simulink model "purePursuitUSCity"  (R2022b)
settings: Solver=VariableStepAuto  StartTime=0.0  StopTime=Ts  RelTol=1e-3
PreLoadFcn:
  | setUpPurePursuitUSCity
model workspace (MAT data in the model file):
  firstWarning = 0
  originalScenarioChecksum = 'F73A6DA3C723D3CA73A6F931B7A52A9C'
values from neighbouring files (symbols this model uses):
  diffcurve = []    [setUpPurePursuitUSCity.m]
  L = data.ActorSpecifications.Length    [setUpPurePursuitUSCity.m]
  ld = 5    [setUpPurePursuitUSCity.m]
  psi_o = refPose(1,3)    [setUpPurePursuitUSCity.m]
  s = size(xRef)    [setUpPurePursuitUSCity.m]
  X_o = refPose(1,1)    [setUpPurePursuitUSCity.m]
  xRef = refPose(:,1)    [setUpPurePursuitUSCity.m]
  Y_o = -refPose(1,2)    [setUpPurePursuitUSCity.m]
  yRef = -refPose(:,2)    [setUpPurePursuitUSCity.m]
undefined symbols (not defined in the file or in its folder): data, deg, rad
libraries: autolibutils x4, autolibshared x3, vehdynlibviscommon x1, aerolibconvert2 x1, simulink_extras x1, drivingscenarioandsensors x1, robotalgslib x1, simulink x1, sim3dlib x1, vdynlib x1
(part 1 of 3)
settings Model: PacingRate=0.700000  Creator=valakshe  LastModifiedBy=burak
settings SolverCC: AlgebraicLoopSolver=TrustRegion
settings DebuggingCC: UnconnectedInputMsg=warning  UnconnectedOutputMsg=warning  UnconnectedLineMsg=warning  SFMachineParentedDataDiag=warning
settings ModelReferenceCC: EnableRefExpFcnMdlSchedulingChecks=on
settings RTWCC: DLArmComputeVersion=19.05

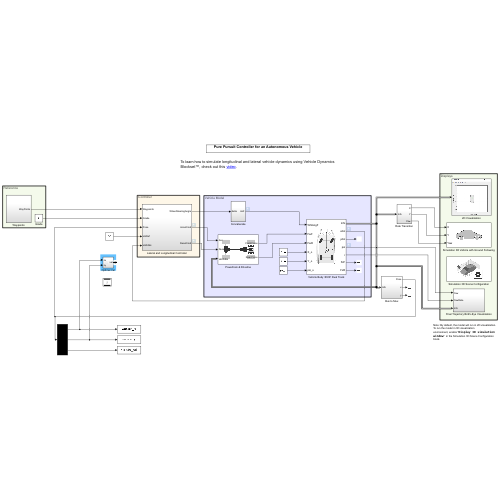
[thumbnail: Simulink's stored preview of the top-level diagram]
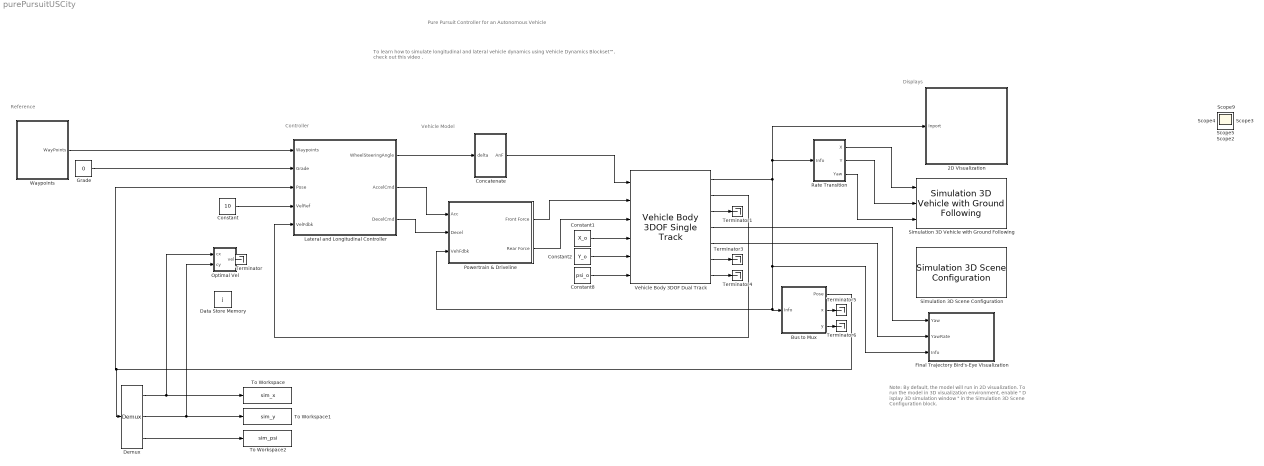
== system purePursuitUSCity ==
  note: Note: By default, the model will run in 2D visualization. To run the model in 3D visualization
      | environment, enable " D isplay 3D simulation window " in the Simulation 3D Scene Configuration block.
  note: To learn how to simulate longitudinal and lateral vehicle dynamics using Vehicle Dynamics
      | Blockset™, check out this video .
  note: Pure Pursuit Controller for an Autonomous Vehicle
  note: Reference
  note: Controller
  note: Vehicle Model
  note: Displays
  2D Visualization : Subsystem
      mask Display: image("visualization.JPG");
  Bus to Mux : Subsystem
  Concatenate : Subsystem
  Constant : Constant  Value=10
  Constant1 : Constant  Value=X_o
  Constant2 : Constant  Value=Y_o
  Constant8 : Constant  Value=psi_o
  Data Store Memory : DataStoreMemory  DataStoreName=j  WriteAfterWriteMsg=warning  InitialValue=j  ShowAdditionalParam=off
  Demux : Demux  Outputs=3
  Final Trajectory Bird's-Eye Visualization : Subsystem
  Grade : Constant  Value=0
  Lateral and Longitudinal Controller : Subsystem
  Optimal Vel : Subsystem
  Powertrain & Driveline : Subsystem
      mask Display: image('vdbslibpt.png');
  Rate Transition : Subsystem
  Simulation 3D Scene Configuration : sim3dlib/Simulation 3D Scene Configuration  Priority=1  ProjectFormat=Default Scenes  SceneDesc=Curved road  ProjectName=C:\Program Files\MATLAB\R2022b\toolbox\shared\sim3d_projects\automotive_project\UE4\WindowsNoEditor\VehicleSimulation.exe  ScenePath=8mile  UEProjPath=C:\Local\AutoVrtlEnv\AutoVrtlEnv.uproject  EnableOpenDRIVE=off  vehTagList={'Scene Origin';'SimulinkVehicle1'}  vehTag=SimulinkVehicle1  OpVisEn=off  Ts=.05  EnableWindow=on  EnableRemoteAccess=off  EnableWeather=off  SunAltitude=40.0  SunAzimuth=90  clouds=10  wind=1  fog=0  rain=0  EnableGeospatial=off  OriginHeight=200  OriginLatitude=40.744652  OriginLongitude=-73.988864  MapStyle=Aerial  AdditionalAssetIDs=[]  UseAdvancedSunSky=off  SolarTime=11  TimeZone=-5  Day=21  Month=9  Year=2022  UseDaylightSavingTime=on  DSTStartDay=10  DSTStartMonth=3  DSTEndDay=3  DSTEndMonth=11  DSTSwitchHour=2  sensorTag=MainCamera1  sensorId=1  sensorName=MainCamera1  mountLoc=Origin  offsetFlag=off  tmountOffset=[0, 0, 0]  rmountOffset=[0, 0, 0]  HorizontalResolution=1280  VerticalResolution=720  HorizontalFOV=60  mountPoint=[0 0 0]  mountOrientation=[0 0 0]  aMode=2  ID=1  GeoTrigger=Inactive
  Simulation 3D Vehicle with Ground Following : vdynlib/Vehicle Scenarios/Sim3D/Sim3D Vehicle/Components/Simulation 3D Vehicle with Ground Following  Priority=-1  PassVehMesh=Muscle car  MeshPath=/MathWorksSimulation/Vehicles/Muscle/Meshes/SK_MuscleCar.SK_MuscleCar  TrackWidth=1.9  WheelBase=3  WheelRadius=0.35  VehColor=Yellow  InitialPos=[0,0,0]  InitialRot=[0, 0, 0]  ActorName=SimulinkVehicle1  VehLightsControl=off  HeadlightColor=[ 1, 1, 1 ]  HighBeamIntensity=100000  LowBeamIntensity=60000  HighBeamConeAngle=1.22  LowBeamConeAngle=1.22  LeftHeadlightOrientation=[ 0, 0 ]  RightHeadlightOrientation=[ 0, 0 ]  BrakelightIntensity=200  ReverselightIntensity=500  SignallightIntensity=500  SignallightPeriod=1  SignalPulseWidth=50  SampleTime=-1  ActorType=SimulinkVehicle  ID=1  aMode=2  ActorTag=SimulinkVehicle1  CoordinateScheme=SAE
  Terminator{,1,3..6} (6 alike) : Terminator
  To Workspace : ToWorkspace  VariableName=sim_x  SaveFormat=Timeseries  SampleTime=-1
  To Workspace1 : ToWorkspace  VariableName=sim_y  SaveFormat=Timeseries  SampleTime=-1
  To Workspace2 : ToWorkspace  VariableName=sim_psi  SaveFormat=Timeseries  SampleTime=-1
  Vehicle Body 3DOF Dual Track : autolibshared/Vehicle Body 3DOF Single Track  trackMode=Dual  inputMode=External longitudinal forces  frontSteerMode=on  rearSteerMode=off  windMode=off  muMode=off  extFMode=off  extMMode=off  htchFMode=off  htchMMode=off  extXo=on  extpsio=on  extxdoto=off  extro=off  extYo=on  extTamb=off  extydoto=off  aMode=2  NF=2  NR=2  m=2000  a=1.4  b=1.6  h=0.35  dh=1  hh=0.2  X_o=0  xdot_o=0  CalphaMode=off  sigmaMode=on  d=0  hl=0  w=[1.4,1.4]  Cy_f=12e3  Cy_r=11e3  sigma_f=.1  sigma_r=.1  alpha_f_brk=[-.1 .1]  Cy_f_data=[-9e3 9e3]  alpha_r_brk=[-.1 .1]  Cy_r_data=[-9e3 9e3]  Y_o=0  ydot_o=0  Izz=4000  psi_o=0  r_o=0  Af=2  Cd=.3  Cl=.1  Cpm=.1  beta_w=[0:0.01:0.3]  Cs=[0:0.03:0.9]  Cym=[0:0.01:0.3]  Pabs=101325  Tair=273  g=9.81  mu=1  xdot_tol=.01  Fznom=5000  Fxtire_sat=7e4  Fytire_sat=7e4  longOff=0  latOff=0  vertOff=0  wrapAng=off
  Waypoints : Subsystem
  Scope{,1..5,9} (7 alike) : Scope
  wires:
  Vehicle Body 3DOF Dual Track/7 -> Terminator4/1
  Vehicle Body 3DOF Dual Track/3 -> Terminator1/1
  Constant1/1 -> Vehicle Body 3DOF Dual Track/4
  Vehicle Body 3DOF Dual Track/6 -> Terminator3/1
  Constant2/1 -> Vehicle Body 3DOF Dual Track/5
  Concatenate/1(AnF) -> Vehicle Body 3DOF Dual Track/1
  Powertrain & Driveline/1(Front Force) -> Vehicle Body 3DOF Dual Track/2
  Powertrain & Driveline/2(Rear Force) -> Vehicle Body 3DOF Dual Track/3
  Constant8/1 -> Vehicle Body 3DOF Dual Track/6
  Vehicle Body 3DOF Dual Track/1 -> 2D Visualization/1(Inport), Rate Transition/1(Info), Powertrain & Driveline/3(VehFdbk), Bus to Mux/1(Info), Final Trajectory Bird's-Eye Visualization/3(Info)
  Lateral and Longitudinal Controller/1(WheelSteeringAngle) -> Concatenate/1(delta)
  Lateral and Longitudinal Controller/2(AccelCmd) -> Powertrain & Driveline/1(Acc)
  Lateral and Longitudinal Controller/3(DecelCmd) -> Powertrain & Driveline/2(Decel)
  Waypoints/1(WayPoints) -> Lateral and Longitudinal Controller/1(Waypoints)
  Grade/1 -> Lateral and Longitudinal Controller/2(Grade)
  Bus to Mux/1(Pose) -> Demux/1, Lateral and Longitudinal Controller/3(Pose)
  Vehicle Body 3DOF Dual Track/2 -> Lateral and Longitudinal Controller/5(VelFdbk)
  Rate Transition/1(X) -> Simulation 3D Vehicle with Ground Following/1
  Rate Transition/2(Y) -> Simulation 3D Vehicle with Ground Following/2
  Rate Transition/3(Yaw) -> Simulation 3D Vehicle with Ground Following/3
  Vehicle Body 3DOF Dual Track/4 -> Final Trajectory Bird's-Eye Visualization/1(Yaw)
  Vehicle Body 3DOF Dual Track/5 -> Final Trajectory Bird's-Eye Visualization/2(YawRate)
  Bus to Mux/2(x) -> Terminator5/1
  Bus to Mux/3(y) -> Terminator6/1
  Demux/3 -> To Workspace2/1
  Demux/2 -> To Workspace1/1, Optimal Vel/2("cy ")
  Demux/1 -> Optimal Vel/1(cx), To Workspace/1
  Optimal Vel/1(vel) -> Terminator/1
  Constant/1 -> Lateral and Longitudinal Controller/4(VelRef)

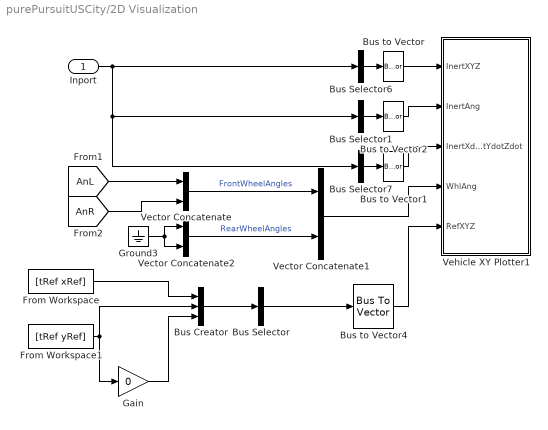
== system purePursuitUSCity/2D Visualization ==
  Inport : Inport
  Bus Creator : BusCreator  Inputs=3
  Bus Selector : BusSelector  OutputSignals=signal1,signal2,signal3  OutputAsBus=on
  Bus Selector1 : BusSelector  OutputSignals=InertFrm.Cg.Ang.phi,InertFrm.Cg.Ang.theta,InertFrm.Cg.Ang.psi  OutputAsBus=on
  Bus Selector6 : BusSelector  OutputSignals=InertFrm.Geom.Disp.X,InertFrm.Geom.Disp.Y,InertFrm.Geom.Disp.Z  OutputAsBus=on
  Bus Selector7 : BusSelector  OutputSignals=InertFrm.Geom.Vel.Xdot,InertFrm.Geom.Vel.Ydot,InertFrm.Geom.Vel.Zdot  OutputAsBus=on
  Bus to Vector{,1..2,4} (4 alike) : BusToVector
  From Workspace : FromWorkspace  VariableName=[tRef xRef]
  From Workspace1 : FromWorkspace  VariableName=[tRef yRef]
  Gain : Gain  Gain=0
  Ground3 : Ground
  Vector Concatenate : Concatenate
  Vector Concatenate1 : Concatenate
  Vector Concatenate2 : Concatenate
  Vehicle XY Plotter1 : Subsystem  mask(Vehicle XY Plotter){extRef=on, extStats=off, extTireF=off, a=2, b=2, w=2, figBorder=10, bufferSize=1024, velNorm=5, tireFNorm=1000, pltDT=0.2}
      mask prompts: extRef "Plot path reference, extRef"; extStats "Display speed, RPM and Gear"; extTireF "Display tire forces"; a "Distance to front axle from CG, a [m]:"; b "Distance to rear axle from CG, b [m]:"; w "Track width, w [m]:"; figBorder "Distance to figure borders, figBorder [m]:"; bufferSize "Path buffer sampe size, bufferSize []:"; velNorm "Velocity vector scaling, velNorm [m*s/m]:"; tireFNorm "Tire force vector scaling, tireFNorm [m/N]:"; pltDT "Plot update rate, pltDT [s]:"
      mask help:
      | This block will display a MATLAB figure which indicates the vehicle path, current position and heading velocity.
      | An optional path reference is also provided.
      mask init:
      | block = gcb;
      | if autoblkschecksimstopped(block)
      |     ParamNames = {'extRef';'extStats';'extTireF';'extTireF'};
      |     PortNames = {'RefXYZ';'Stats';'TireFx';'TireFy'};
      |     for idx=1:length(PortNames)
      |         InportOption  = {'built-in/Ground', [PortNames{idx}, ' Ground'];...
      |             'built-in/Inport',PortNames{idx}};
      |         if ~strcmp(get_param(block,ParamNames{idx}),'on')
      |             NewBlkHdl = autoblksreplaceblock(block, InportOption, 1);
      |             set_param(NewBlkHdl, 'ShowName', 'off');
      |         else
      |             autoblksreplaceblock(block, InportOption, 2);
      |         end
      |     end
      |     InportNames = {'InertXYZ';'InertAng';'InertXdotYdotZdot';'WhlAng';'RefXYZ';'Stats';'TireFx';'TireFy'};
      |     FoundNames = get_param(find_system(block, 'LookUnderMasks', 'all', 'SearchDepth', 1, 'FollowLinks', 'on', 'BlockType', 'Inport'), 'Name');
      |     [~,PortI] = intersect(InportNames, FoundNames);
      |     PortI = sort(PortI);
      |     for idx = 1:length(PortI)
      |         set_param([block, '/', InportNames{PortI(idx)}], 'Port', num2str(idx));
      |     end
      | end
      mask TypeOptions a: Vehicle XY Plotter/a
      mask TypeOptions b: Vehicle XY Plotter/b
      mask TypeOptions w: Vehicle XY Plotter/w
      mask TypeOptions figBorder: Vehicle XY Plotter/figBorder
      mask TypeOptions bufferSize: Vehicle XY Plotter/bufferSize
      mask TypeOptions velNorm: Vehicle XY Plotter/velNorm
      mask TypeOptions tireFNorm: Vehicle XY Plotter/tireFNorm
      mask DialogControl Container3 Prompt: Plot and Display Options
  wires:
  Vector Concatenate1/1 -> Vehicle XY Plotter1/4(WhlAng)
  Ground3/1 -> Vector Concatenate2/1, Vector Concatenate2/2
  Bus Selector6/1 -> Bus to Vector/1
  Vector Concatenate/1 -> Vector Concatenate1/1  "FrontWheelAngles"
  [AnL] -> Vector Concatenate/1
  Vector Concatenate2/1 -> Vector Concatenate1/2  "RearWheelAngles"
  Bus Selector7/1 -> Bus to Vector1/1
  Bus to Vector1/1 -> Vehicle XY Plotter1/3(InertXdotYdotZdot)
  Bus to Vector/1 -> Vehicle XY Plotter1/1(InertXYZ)
  Bus to Vector2/1 -> Vehicle XY Plotter1/2(InertAng)
  Bus Selector1/1 -> Bus to Vector2/1
  [AnR] -> Vector Concatenate/2
  Inport/1 -> Bus Selector7/1, Bus Selector1/1, Bus Selector6/1
  Bus to Vector4/1 -> Vehicle XY Plotter1/5(RefXYZ)
  Bus Selector/1 -> Bus to Vector4/1
  From Workspace1/1 -> Gain/1, Bus Creator/2
  Gain/1 -> Bus Creator/3
  From Workspace/1 -> Bus Creator/1
  Bus Creator/1 -> Bus Selector/1

== system purePursuitUSCity/Bus to Mux ==
  Info : Inport
  Bus Selector1 : BusSelector  OutputSignals=InertFrm.Cg.Disp.X,InertFrm.Cg.Disp.Y,InertFrm.Cg.Ang.psi
  Mux : Mux  Inputs=3
  Pose : Outport
  x : Outport  Port=2
  y : Outport  Port=3
  wires:
  Bus Selector1/3 -> Mux/3  "<psi>"
  Bus Selector1/1 -> Mux/1, x/1  "<X>"
  Mux/1 -> Pose/1
  Bus Selector1/2 -> y/1, Mux/2  "<Y>"
  Info/1 -> Bus Selector1/1

== system purePursuitUSCity/Concatenate ==
  delta : Inport
  Matrix Concatenate : Concatenate
  AnF : Outport  VectorParamsAs1DForOutWhenUnconnected=off
  tag scope: AnL=global, AnR=global
  wires:
  Matrix Concatenate/1 -> AnF/1
  delta/1 -> [AnL], [AnR], Matrix Concatenate/2, Matrix Concatenate/1

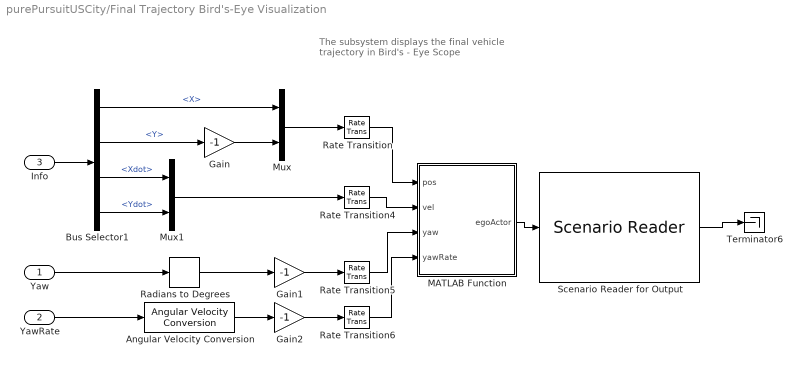
== system purePursuitUSCity/Final Trajectory Bird's-Eye Visualization ==
  note: The subsystem displays the final vehicle trajectory in Bird's - Eye Scope
  Yaw : Inport
  YawRate : Inport  Port=2
  Info : Inport  Port=3
  Angular Velocity Conversion : aerolibconvert2/Angular Velocity Conversion  IU=rad/s  OU=deg/s
  Bus Selector1 : BusSelector  OutputSignals=InertFrm.Cg.Disp.X,InertFrm.Cg.Disp.Y,InertFrm.Cg.Vel.Xdot,InertFrm.Cg.Vel.Ydot
  Gain : Gain  Gain=-1
  Gain1 : Gain  Gain=-1
  Gain2 : Gain  Gain=-1
  MATLAB Function : MATLAB Function  TreatAsAtomicUnit=on
  Mux : Mux  Inputs=2
  Mux1 : Mux  Inputs=2
  Radians to Degrees : simulink_extras/Transformations/Radians to Degrees
  Rate Transition{,4..6} (4 alike) : RateTransition
  "Scenario Reader for Output " : drivingscenarioandsensors/Scenario Reader  ScenarioSource=From file  ScenarioFileName=USCity.mat  ScenarioVariableName=scenario  OutputCoordinateSystem=Vehicle coordinates  EgoVehicleSource=Input port  EgoVehicleActorID=1  OrientVehiclesOnRoad=off  OutputEgoVehiclePose=on  OutputEgoVehicleState=off  SampleTime=0.1  LaneBoundaryOutput=None  LaneBoundaryDistance=0:0.5:9.5  LaneBoundaryLocation=Center of lane markings  BusNameSource=Property  BusName=BusActors  BusNumActorsSource=Scenario  BusNumActors=100  BusName2Source=Auto  BusName2=BusLaneBoundaries  BusNumLaneBoundariesSource=Scenario  BusNumLaneBoundaries=10  BusName3Source=Auto  BusName3=BusEgoActor  BusName4Source=Auto  BusName4=BusEgoState  ShowCoordinateLabels=on  SimulateUsing=Interpreted execution
  Terminator6 : Terminator
  wires:
  "Scenario Reader for Output "/1 -> Terminator6/1
  YawRate/1 -> Angular Velocity Conversion/1
  Yaw/1 -> Radians to Degrees/1
  Gain2/1 -> Rate Transition6/1
  Gain1/1 -> Rate Transition5/1
  Angular Velocity Conversion/1 -> Gain2/1
  Radians to Degrees/1 -> Gain1/1
  Info/1 -> Bus Selector1/1
  Bus Selector1/3 -> Mux1/1  "<Xdot>"
  Mux/1 -> Rate Transition/1
  Gain/1 -> Mux/2
  Bus Selector1/4 -> Mux1/2  "<Ydot>"
  Rate Transition5/1 -> MATLAB Function/3(yaw)
  Mux1/1 -> Rate Transition4/1
  MATLAB Function/1(egoActor) -> "Scenario Reader for Output "/1
  Rate Transition4/1 -> MATLAB Function/2(vel)
  Bus Selector1/2 -> Gain/1  "<Y>"
  Bus Selector1/1 -> Mux/1  "<X>"
  Rate Transition/1 -> MATLAB Function/1(pos)
  Rate Transition6/1 -> MATLAB Function/4(yawRate)

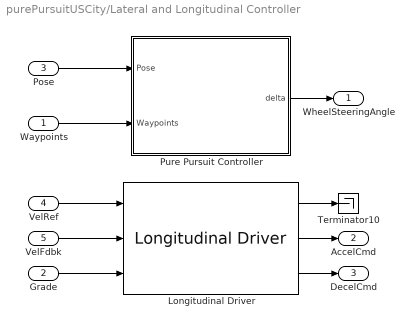
== system purePursuitUSCity/Lateral and Longitudinal Controller ==
  Waypoints : Inport
  Grade : Inport  Port=2
  Pose : Inport  Port=3
  VelRef : Inport  Port=4
  VelFdbk : Inport  Port=5
  Longitudinal Driver : autolibshared/Longitudinal Driver  extAccelOvr=off  extDecelOvr=off  extAccelHld=off  extDecelHld=off  extAccelZero=off  extDecelZero=off  cntrlType=PI  shftType=None  velUnits=m/s  gearOut=off  Kp=100  Ki=1  Kff=.1  Kg=0  VehVelVec=[0 100]  KffVec=[.1 .1]  KpVec=[10 10]  KiVec=[5 5]  KgVec=[0 0]  m=1500  Kpt=3000  tau=.1  L=2  aR=200  bR=2.5  cR=.5  g=9.81  vnom=9  Kaw=1  tauerr=.01  tauPt=2  GearInit=0  tShift=.1  pdlVec=[0.1 0.4 0.5 0.9]  upShftTbl=[-1 12.9375 26.4375 39.9375 51.18749999999999 62.4375 72.84375 83.25;-1 16.3125 29.8125 43.3125 54.5624 65.8125 76.78125 87.75;-1 19.6875 33.1875 46.68749999999999 57.9375 69.1875 80.71875 92.25;-1 33 52.5 77.25 100.5 138.75 161.875 185]  dwnShftTbl=[1 9.5625 23.0625 36.5625 47.8125 59.0625 68.90625 78.75;1 12.9375 26.4375 39.9375 51.18749999999999 62.4375 72.84375 83.25;1 16.3125 29.8125 43.3125 54.562499 65.8125 76.78125 87.75;1 19.6875 33.1875 46.68749999999999 57.9375 69.1875 80.71875 92.25]  tClutch=.5  tRev=.5  tPark=120  aMode=2  UpGearVec="[0  1  2  3  4  5  6  7]"  DownGearVec="[1  2  3  4  5  6  7  8]"
  Pure Pursuit Controller : Subsystem
  Terminator10 : Terminator
  WheelSteeringAngle : Outport
  AccelCmd : Outport  Port=2
  DecelCmd : Outport  Port=3
  wires:
  Pure Pursuit Controller/1(delta) -> WheelSteeringAngle/1
  Waypoints/1 -> Pure Pursuit Controller/2(Waypoints)
  Pose/1 -> Pure Pursuit Controller/1(Pose)
  Grade/1 -> Longitudinal Driver/3
  Longitudinal Driver/3 -> DecelCmd/1
  VelRef/1 -> Longitudinal Driver/1
  VelFdbk/1 -> Longitudinal Driver/2
  Longitudinal Driver/2 -> AccelCmd/1
  Longitudinal Driver/1 -> Terminator10/1

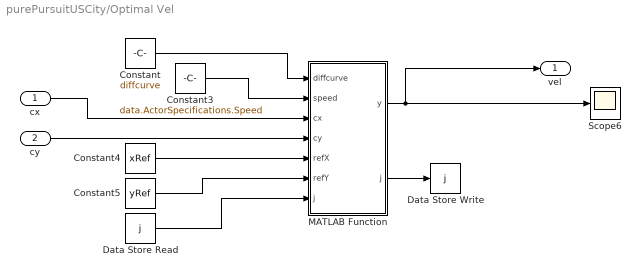
== system purePursuitUSCity/Optimal Vel ==
  cx : Inport
  "cy " : Inport  Port=2
  Constant : Constant  Value=diffcurve
  Constant3 : Constant  Value=data.ActorSpecifications.Speed
  Constant4 : Constant  Value=xRef
  Constant5 : Constant  Value=yRef
  Data Store Read : DataStoreRead  DataStoreName=j  IndexOptions=Index vector (dialog)  Indices=1  OutputSizes=1
  Data Store Write : DataStoreWrite  DataStoreName=j  IndexOptions=Index vector (dialog)  Indices=1  OutputSizes=1
  MATLAB Function : MATLAB Function  TreatAsAtomicUnit=on
  Scope6 : Scope
  vel : Outport
  wires:
  cx/1 -> MATLAB Function/3(cx)
  "cy "/1 -> MATLAB Function/4(cy)
  Constant4/1 -> MATLAB Function/5(refX)
  MATLAB Function/1(y) -> vel/1, Scope6/1
  Constant5/1 -> MATLAB Function/6(refY)
  MATLAB Function/2(j) -> Data Store Write/1
  Data Store Read/1 -> MATLAB Function/7("j ")
  Constant3/1 -> MATLAB Function/2(speed)
  Constant/1 -> MATLAB Function/1(diffcurve)

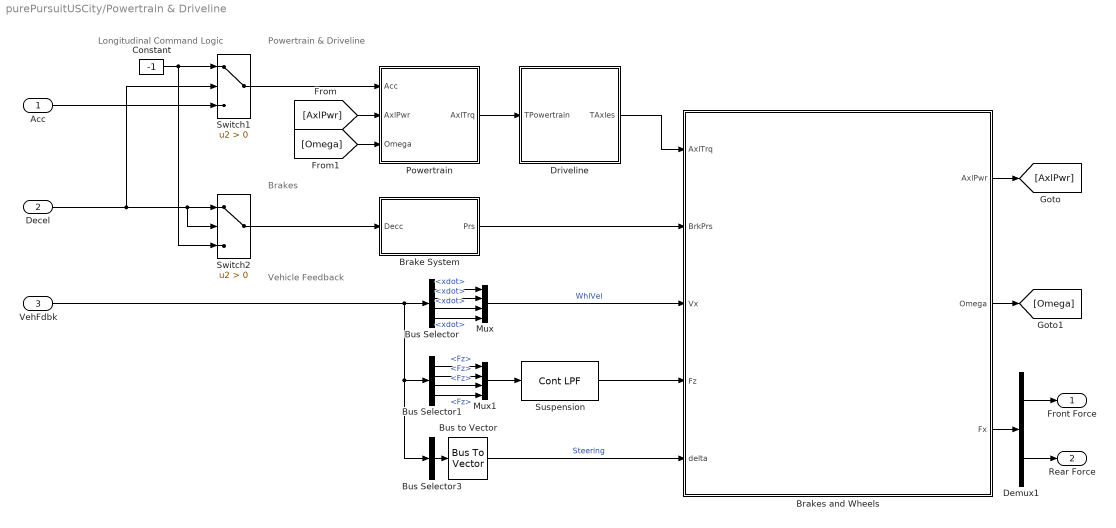
== system purePursuitUSCity/Powertrain & Driveline ==
  note: Vehicle Feedback
  note: Powertrain & Driveline
  note: Brakes
  note: Longitudinal Command Logic
  Acc : Inport
  Decel : Inport  Port=2
  VehFdbk : Inport  Port=3
  Brake System : Subsystem
  Brakes and Wheels : Subsystem  TreatAsAtomicUnit=on
      mask Display: image('vdbslibwhls.png');
  Bus Selector : BusSelector  OutputSignals=BdyFrm.FrntAxl.Lft.Vel.xdot,BdyFrm.FrntAxl.Rght.Vel.xdot,BdyFrm.RearAxl.Lft.Vel.xdot,BdyFrm.RearAxl.Rght.Vel.xdot
  Bus Selector1 : BusSelector  OutputSignals=BdyFrm.Forces.FrntAxl.Lft.Fz,BdyFrm.Forces.FrntAxl.Rght.Fz,BdyFrm.Forces.RearAxl.Lft.Fz,BdyFrm.Forces.RearAxl.Rght.Fz
  Bus Selector3 : BusSelector  OutputSignals=BdyFrm.FrntAxl.Steer.WhlAngFL,BdyFrm.FrntAxl.Steer.WhlAngFR,BdyFrm.RearAxl.Steer.WhlAngRL,BdyFrm.RearAxl.Steer.WhlAngRR  OutputAsBus=on
  Bus to Vector : BusToVector
  Constant : Constant  Value=-1
  Demux1 : Demux  Outputs=[2 2]
  Driveline : Subsystem  Variant=on  VariantControlMode=label  VariantControl=Variant1  LabelModeActiveChoice=0
  Mux : Mux
  Mux1 : Mux
  Powertrain : Subsystem
  Suspension : autolibutils/Cont LPF  wc=10*pi*2  AbsoluteTolerance=auto  aMode=2
  Switch1 : Switch  Criteria=u2 > Threshold  SaturateOnIntegerOverflow=off  InputSameDT=off
  Switch2 : Switch  Criteria=u2 > Threshold  SaturateOnIntegerOverflow=off  InputSameDT=off
  Front Force : Outport  VectorParamsAs1DForOutWhenUnconnected=off
  Rear Force : Outport  Port=2  VectorParamsAs1DForOutWhenUnconnected=off
  wires:
  Brake System/1(Prs) -> Brakes and Wheels/2(BrkPrs)
  Switch2/1 -> Brake System/1(Decc)
  [Omega] -> Powertrain/3(Omega)
  [AxlPwr] -> Powertrain/2(AxlPwr)
  Brakes and Wheels/2(Omega) -> [Omega]
  Powertrain/1(AxlTrq) -> Driveline/1(TPowertrain)
  Switch1/1 -> Powertrain/1(Acc)
  Bus Selector1/4 -> Mux1/4  "<Fz>"
  Bus Selector1/3 -> Mux1/3  "<Fz>"
  Bus Selector1/2 -> Mux1/2  "<Fz>"
  Bus Selector1/1 -> Mux1/1  "<Fz>"
  Bus Selector/4 -> Mux/4  "<xdot>"
  Bus Selector/3 -> Mux/3  "<xdot>"
  Bus Selector/2 -> Mux/2  "<xdot>"
  Bus Selector/1 -> Mux/1  "<xdot>"
  Suspension/1 -> Brakes and Wheels/4(Fz)
  Mux1/1 -> Suspension/1
  Bus to Vector/1 -> Brakes and Wheels/5(delta)  "Steering"
  Bus Selector3/1 -> Bus to Vector/1
  Brakes and Wheels/3(Fx) -> Demux1/1
  Brakes and Wheels/1(AxlPwr) -> [AxlPwr]
  Driveline/1(TAxles) -> Brakes and Wheels/1(AxlTrq)
  Demux1/2 -> Rear Force/1
  Demux1/1 -> Front Force/1
  VehFdbk/1 -> Bus Selector/1, Bus Selector1/1, Bus Selector3/1
  Mux/1 -> Brakes and Wheels/3(Vx)  "WhlVel"
  Constant/1 -> Switch1/1, Switch2/3
  Acc/1 -> Switch1/3
  Decel/1 -> Switch2/1, Switch2/2, Switch1/2

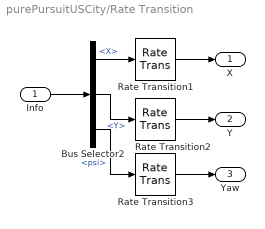
== system purePursuitUSCity/Rate Transition ==
  Info : Inport
  Bus Selector2 : BusSelector  OutputSignals=InertFrm.Geom.Disp.X,InertFrm.Geom.Disp.Y,InertFrm.Cg.Ang.psi
  Rate Transition1 : RateTransition  InitialCondition=X_o  OutPortSampleTime=0.01
  Rate Transition2 : RateTransition  InitialCondition=Y_o  OutPortSampleTime=0.01
  Rate Transition3 : RateTransition  OutPortSampleTime=0.01
  X : Outport
  Y : Outport  Port=2
  Yaw : Outport  Port=3
  wires:
  Info/1 -> Bus Selector2/1
  Rate Transition3/1 -> Yaw/1
  Rate Transition2/1 -> Y/1
  Rate Transition1/1 -> X/1
  Bus Selector2/1 -> Rate Transition1/1  "<X>"
  Bus Selector2/3 -> Rate Transition3/1  "<psi>"
  Bus Selector2/2 -> Rate Transition2/1  "<Y>"

== system purePursuitUSCity/Waypoints ==
  Constant3 : Constant  Value=xRef  SampleTime=0.1
  Constant4 : Constant  Value=yRef  SampleTime=0.1
  Matrix Concatenate : Concatenate  Mode=Multidimensional array  ConcatenateDimension=2
  WayPoints : Outport
  wires:
  Constant4/1 -> Matrix Concatenate/2
  Constant3/1 -> Matrix Concatenate/1
  Matrix Concatenate/1 -> WayPoints/1

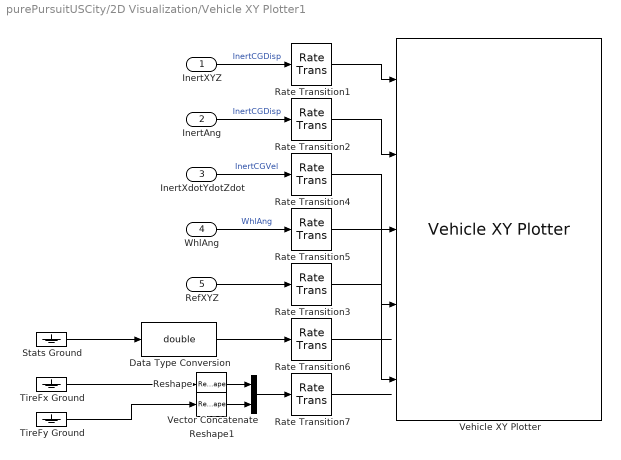
== system purePursuitUSCity/2D Visualization/Vehicle XY Plotter1 ==
  InertXYZ : Inport
  InertAng : Inport  Port=2
  InertXdotYdotZdot : Inport  Port=3
  WhlAng : Inport  Port=4
  RefXYZ : Inport  Port=5
  Data Type Conversion : DataTypeConversion  OutDataTypeStr=double  SaturateOnIntegerOverflow=off  RndMeth=Floor
  Rate Transition{1..7} (7 alike) : RateTransition  Deterministic=off  OutPortSampleTime=pltDT
  Reshape : Reshape  OutputDimensionality=Row vector (2-D)
  Reshape1 : Reshape  OutputDimensionality=Row vector (2-D)
  Stats Ground : Ground
  TireFx Ground : Ground
  TireFy Ground : Ground
  Vector Concatenate : Concatenate  Mode=Multidimensional array
  Vehicle XY Plotter : vehdynlibviscommon/Vehicle XY Plotter  w=w  a=a  b=b  figBorder=figBorder  bufferSize=bufferSize  extStats=off  extTireF=off
  wires:
  Vector Concatenate/1 -> Rate Transition7/1
  Reshape1/1 -> Vector Concatenate/2
  Reshape/1 -> Vector Concatenate/1
  RefXYZ/1 -> Rate Transition3/1
  Rate Transition7/1 -> ?
  Data Type Conversion/1 -> Rate Transition6/1
  Rate Transition6/1 -> ?
  Rate Transition5/1 -> Vehicle XY Plotter/4
  Rate Transition4/1 -> Vehicle XY Plotter/3
  Rate Transition2/1 -> Vehicle XY Plotter/2
  Rate Transition1/1 -> Vehicle XY Plotter/1
  Rate Transition3/1 -> Vehicle XY Plotter/5
  WhlAng/1 -> Rate Transition5/1  "WhlAng"
  InertXYZ/1 -> Rate Transition1/1  "InertCGDisp"
  InertXdotYdotZdot/1 -> Rate Transition4/1  "InertCGVel"
  InertAng/1 -> Rate Transition2/1  "InertCGDisp"
  Stats Ground/1 -> Data Type Conversion/1
  TireFx Ground/1 -> Reshape/1
  TireFy Ground/1 -> Reshape1/1

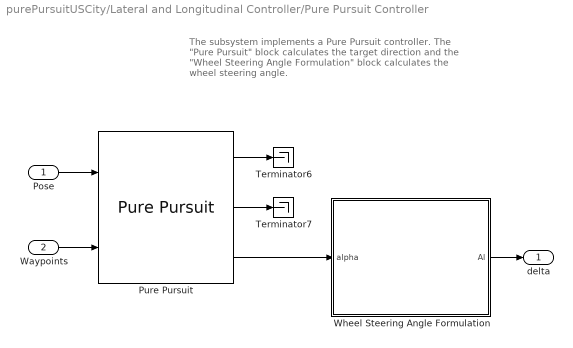
== system purePursuitUSCity/Lateral and Longitudinal Controller/Pure Pursuit Controller ==
  note: The subsystem implements a Pure Pursuit controller. The "Pure Pursuit" block calculates the target direction and the "Wheel Steering Angle Formulation" block calculates the wheel steering angle.
  Pose : Inport
  Waypoints : Inport  Port=2
  Pure Pursuit : robotalgslib/Pure Pursuit  DesiredLinearVelocity=0.1  MaxAngularVelocity=1.0  LookaheadDistance=ld  TargetDirPort=on  SimulateUsing=Code generation
  Terminator6 : Terminator
  Terminator7 : Terminator
  Wheel Steering Angle Formulation : Subsystem  mask{L=L, ld=ld}
      mask prompts: L "Bicycle length"; ld "Lookahead distance"
      mask TypeOptions L: Bicycle length/Value
      mask TypeOptions ld: Lookahead distance/Value
      mask Display:
      | image("GeometryMask.png")
      | port_label('input', 1, 'alpha')
      | port_label('output', 1, 'delta')
  delta : Outport
  wires:
  Wheel Steering Angle Formulation/1(Al) -> delta/1
  Pure Pursuit/3 -> Wheel Steering Angle Formulation/1(alpha)
  Waypoints/1 -> Pure Pursuit/2
  Pure Pursuit/2 -> Terminator7/1
  Pose/1 -> Pure Pursuit/1
  Pure Pursuit/1 -> Terminator6/1

== system purePursuitUSCity/Powertrain & Driveline/Brake System ==
  Decc : Inport
  Hydraulics : autolibutils/Cont LPF  wc=30*pi*2  AbsoluteTolerance=auto  aMode=2
  Pressure : Gain  Gain=2e7
  Saturation1 : Saturate  UpperLimit=inf  LowerLimit=0  ZeroCross=off
  Selector : Selector  InputPortWidth=1  IndexOptions=Index vector (dialog)  Indices=[1 1 1 1]  OutputSizes=1
  Signal Specification : SignalSpecification  Unit=Pa
  Prs : Outport  VectorParamsAs1DForOutWhenUnconnected=off
  wires:
  Signal Specification/1 -> Prs/1
  Decc/1 -> Saturation1/1
  Selector/1 -> Signal Specification/1
  Saturation1/1 -> Hydraulics/1
  Hydraulics/1 -> Pressure/1
  Pressure/1 -> Selector/1
